simulink model "lab3_zadanie1_model"  (R2020b)
settings: Solver=VariableStepAuto  StartTime=0.0  StopTime=10.0  RelTol=1e-3
values from neighbouring files (symbols this model uses):
  y_input = [ a, 0, 0, 0]    [lab3_zadanie1.m]
settings Model: Creator=student  LastModifiedBy=student

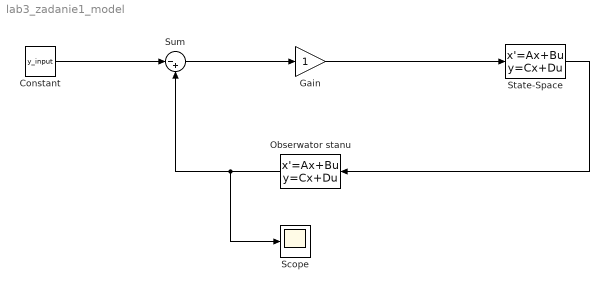
== system lab3_zadanie1_model ==
  Constant : Constant  Value=y_input
  Gain : Gain
  Obserwator stanu : StateSpace  InitialCondition=0
  Scope : Scope
  State-Space : StateSpace  InitialCondition=0
  Sum : Sum  Inputs=|-+
  wires:
  Gain/1 -> State-Space/1
  Sum/1 -> Gain/1
  Constant/1 -> Sum/1
  State-Space/1 -> Obserwator stanu/1
  Obserwator stanu/1 -> Scope/1, Sum/2
